simulink model "Compensator"  (R2024b)
settings: Solver=VariableStepAuto  StartTime=0.0  StopTime=10.0  RelTol=1e-3
libraries: simulink_extras x5, slctrl_linear x2
settings Model: Creator=TC63  LastModifiedBy=TC63

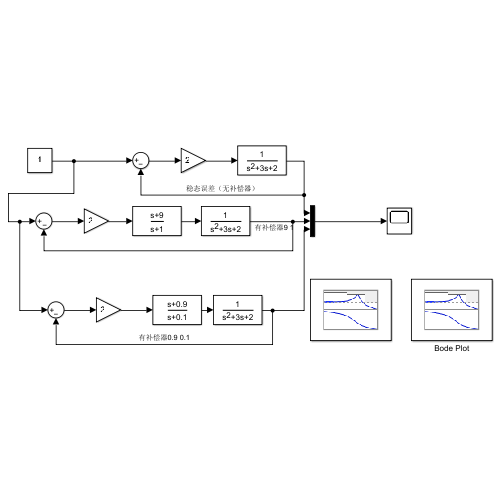
[thumbnail: Simulink's stored preview of the top-level diagram]
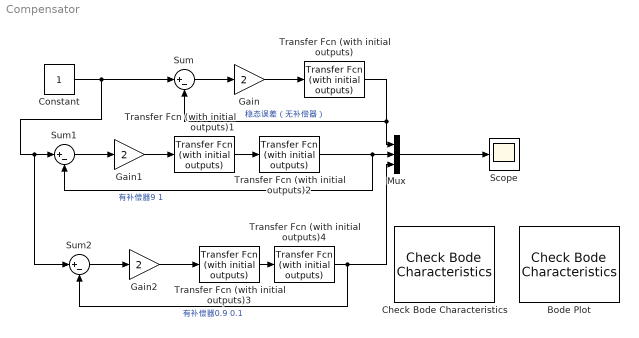
== system Compensator ==
  Bode Plot : slctrl_linear/Check Bode  Characteristics  InstantiateOnLoad=on  SaveOperatingPoints=off  LinearizationIOs={}  LinearizeAt=SnapshotTimes  SnapshotTimes=[0]  TriggerType=rising  SampleTime=auto  RateConversionMethod=zoh  PreWarpFreq=10  UseExactDelayModel=off  UseFullBlockNameLabels=off  UseBusSignalLabels=off  enabled=on  stopWhenAssertionFail=off  export=off  ViewDlgPos=[100 199.666666666667 510 390]  OpenViewOnLoad=off  LaunchViewOnOpen=off  FrequencyUnits=rad/s  MagnitudeUnits=dB  PhaseUnits=deg  TimeUnits=seconds  EnableUpperBound=off  UpperBoundFrequencies=[]  UpperBoundMagnitudes=[]  EnableLowerBound=off  LowerBoundFrequencies=[]  LowerBoundMagnitudes=[]
      settings: LibrarySourceBlock=slctrlblks/Linear Analysis Plots/Bode Plot  SaveToWorkspace=off  SaveName=sys
  Check Bode Characteristics : slctrl_linear/Check Bode  Characteristics  InstantiateOnLoad=on  SaveOperatingPoints=off  LinearizationIOs={}  LinearizeAt=SnapshotTimes  SnapshotTimes=[0]  TriggerType=rising  SampleTime=auto  RateConversionMethod=zoh  PreWarpFreq=10  UseExactDelayModel=off  UseFullBlockNameLabels=off  UseBusSignalLabels=off  enabled=on  stopWhenAssertionFail=off  export=off  ViewDlgPos=[]  OpenViewOnLoad=off  LaunchViewOnOpen=on  FrequencyUnits=rad/s  MagnitudeUnits=dB  PhaseUnits=deg  TimeUnits=seconds  EnableUpperBound=on  UpperBoundFrequencies=[10 100]  UpperBoundMagnitudes=[-20 -20]  EnableLowerBound=on  LowerBoundFrequencies=[0.1 1]  LowerBoundMagnitudes=[20 20]
      settings: SaveToWorkspace=off  SaveName=sys
      settings: LibrarySourceBlock=|
      | slctrlblks/Model Verification/Check Bode
      | Characteristics
  Constant : Constant
  Gain : Gain  Gain=2
  Gain1 : Gain  Gain=2
  Gain2 : Gain  Gain=2
  Mux : Mux  Inputs=3
  Scope : Scope
  Sum : Sum  Inputs=|+-
  Sum1 : Sum  Inputs=|+-
  Sum2 : Sum  Inputs=|+-
  Transfer Fcn (with initial outputs) : simulink_extras/Additional Linear/Transfer Fcn (with initial outputs)  N=[1]  D=[1 3 2]  Y0=0  U0=0
  Transfer Fcn (with initial outputs)1 : simulink_extras/Additional Linear/Transfer Fcn (with initial outputs)  N=[1 9]  D=[1 1]  Y0=0  U0=0
  Transfer Fcn (with initial outputs)2 : simulink_extras/Additional Linear/Transfer Fcn (with initial outputs)  N=[1]  D=[1 3 2]  Y0=0  U0=0
  Transfer Fcn (with initial outputs)3 : simulink_extras/Additional Linear/Transfer Fcn (with initial outputs)  N=[1 0.9]  D=[1 0.1]  Y0=0  U0=0
  Transfer Fcn (with initial outputs)4 : simulink_extras/Additional Linear/Transfer Fcn (with initial outputs)  N=[1]  D=[1 3 2]  Y0=0  U0=0
  wires:
  Gain/1 -> Transfer Fcn (with initial outputs)/1
  Sum/1 -> Gain/1
  Transfer Fcn (with initial outputs)/1 -> Mux/1, Sum/2  "稳态误差（无补偿器）"
  Constant/1 -> Sum2/1, Sum1/1, Sum/1
  Mux/1 -> Scope/1
  Gain1/1 -> Transfer Fcn (with initial outputs)1/1
  Sum1/1 -> Gain1/1
  Transfer Fcn (with initial outputs)2/1 -> Sum1/2, Mux/2  "有补偿器9 1"
  Transfer Fcn (with initial outputs)1/1 -> Transfer Fcn (with initial outputs)2/1
  Transfer Fcn (with initial outputs)3/1 -> Transfer Fcn (with initial outputs)4/1
  Transfer Fcn (with initial outputs)4/1 -> Mux/3, Sum2/2  "有补偿器0.9 0.1"
  Gain2/1 -> Transfer Fcn (with initial outputs)3/1
  Sum2/1 -> Gain2/1
